simulink model "warplab_mimo_4x4"  (Simulink 6.5)
settings: Solver=ode45  StartTime=0.0  StopTime=20000  RelTol=1e-3
undefined symbols (not defined in the file): gcbh, xlBlockLoadCallback
libraries: xbsIndex_r4 x188
(part 4 of 17)

== system warplab_mimo_4x4/Radio_1 Tx_Buffer ==
  RdAddr : Inport
  Rst : Inport  Port=2
  En : Inport  Port=3
  Constant2_SMWOAddr_TxBuff_Radio1_SMWODataI_TxBuff_Radio1_SMWOWE_TxBuff_Radio1 : Constant  Value=0  OutDataType=sfix(16)  ConRadixGroup=Use specified scaling  OutScaling=2^0  SampleTime=inf  FramePeriod=inf
  Constant3 : S-Function  LoadFcn=xlBlockLoadCallback(gcbh);  FunctionName=sysgen  Parameters=ptable_  mask(Xilinx Constant Block Block){arith_type_sgadvanced=, arith_type=Unsigned, const=0, n_bits=32, bin_pt=0, explicit_period_sgadvanced=, explicit_period=off, period=1, dsp48_infoedit=The use of this block for DSP48 instructions is deprecated.  Please use the Opmode block., equ=P=C, opselect_sgadvanced=, opselect=C, inp2_sgadvanced=, inp2=PCIN>>17, opr_sgadvanced=, opr=+, inp1_sgadvanced=, inp1=P, carry_sgadvanced=, carry=CIN, dbl_ovrd_sgadvanced=, dbl_ovrd=off, has_advanced_control=0, sggui_pos=-1,-1,-1,-1, block_type=constant, block_version=VER_STRING_GOES_HERE, sg_icon_stat=25,18,0,1,white,blue,0,c7c04a0c, sg_mask_display=|, sg_list_contents=, sg_blockgui_xml=}
      mask sg_mask_display=|
      | fprintf('','COMMENT: begin icon graphics');
      | patch([0 55 55 0 ],[0 0 26 26 ],[0.77 0.82 0.91]);
      | patch([20 16 22 16 20 27 29 31 38 32 26 22 28 22 26 32 38 31 29 27 20 ],[3 7 13 19 23 23 21 23 23 17 23 19 13 7 3 9 3 3 5 3 3 ],[0.98 0.96 0.92]);
      | plot([0 0 55 55 0 ],[0 26 26 0 0 ]);
      | fprintf('','COMMENT: end icon graphics');
      | fprintf('','COMMENT: begin icon text');
      | color('black');port_label('output',1,'0');
      | fprintf('','COMMENT: end icon text');
      mask prompts: arith_type_sgadvanced ""; arith_type "Type"; const "Constant value"; n_bits "Number of bits"; bin_pt "Binary point"; explicit_period_sgadvanced ""; explicit_period "Sampled constant"; period "Sample period"; dsp48_infoedit ""; equ "DSP48 operation"; opselect_sgadvanced ""; opselect "Operation select"; inp2_sgadvanced ""; inp2 "Z mux"; opr_sgadvanced ""; opr "Operand"; inp1_sgadvanced ""; inp1 "YX muxes"; carry_sgadvanced ""; carry "Carry input"; dbl_ovrd_sgadvanced ""; dbl_ovrd "Override with doubles"; has_advanced_control ""; sggui_pos ""; block_type ""; block_version ""; sg_icon_stat ""; sg_mask_display ""; sg_list_contents ""; sg_blockgui_xml ""
      mask help: Xilinx Constant Block
      mask init: same as warplab_mimo_4x4/CaptureDone/zero3
      settings: CopyFcn=xlBlockMoveCallback(gcbh);  DeleteFcn=xlDestroyGui(gcbh);  ModelCloseFcn=xlDestroyGui(gcbh);  PreSaveFcn=xlBlockPreSaveCallback(gcbh);  PostSaveFcn=xlBlockPostSaveCallback(gcbh);  DestroyFcn=xlDestroyGui(gcbh);  OpenFcn=xlOpenGui(gcbh, 'constant_gui.xml', @constantenablement, @constantaction)  CloseFcn=xlDestroyGui(gcbh);  MoveFcn=xlBlockMoveCallback(gcbh);
      mask Help: eval('xlWeb(xlhtmldoclink(''Constant''))');
      mask StyleString: edit,popup(Boolean|Signed (2's comp)|Unsigned|DSP48 Instruction),edit,edit,edit,edit,checkbox,edit,edit,edit,edit,popup(C + A*B|PCIN + A*B|P + A*B|A * B|C + A:B|C - A:B|C|Custom),edit,popup(0|PCIN|P|C|PCIN>>17|P>>17),edit,popup(+|-),edit,popup(0|P|A:B|A*B|C|P+C|A:B+C),edit,popup(0|1|CIN|~SIGN(P or PCIN)|~SIGN(A*B or A:B)|~SIGND(A*B or A:B)),edit,checkbox,edit,edit,edit,edit,edit,edit,edit,edit
      mask Display:
      | fprintf('','COMMENT: begin icon graphics');
      | patch([0 55 55 0 ],[0 0 26 26 ],[0.77 0.82 0.91]);
      | patch([20 16 22 16 20 27 29 31 38 32 26 22 28 22 26 32 38 31 29 27 20 ],[3 7 13 19 23 23 21 23 23 17 23 19 13 7 3 9 3 3 5 3 3 ],[0.98 0.96 0.92]);
      | plot([0 0 55 55 0 ],[0 26 26 0 0 ]);
      | fprintf('','COMMENT: end icon graphics');
      | fprintf('','COMMENT: begin icon text');
      | color('black');port_label('output',1,'0');
      | fprintf('','COMMENT: end icon text');
  Constant4 : S-Function  LoadFcn=xlBlockLoadCallback(gcbh);  FunctionName=sysgen  Parameters=ptable_  mask(Xilinx Constant Block Block){arith_type_sgadvanced=, arith_type=Boolean, const=0, n_bits=1, bin_pt=0, explicit_period_sgadvanced=, explicit_period=off, period=1, dsp48_infoedit=The use of this block for DSP48 instructions is deprecated.  Please use the Opmode block., equ=P=C, opselect_sgadvanced=, opselect=C, inp2_sgadvanced=, inp2=PCIN>>17, opr_sgadvanced=, opr=+, inp1_sgadvanced=, inp1=P, carry_sgadvanced=, carry=CIN, dbl_ovrd_sgadvanced=, dbl_ovrd=off, has_advanced_control=0, sggui_pos=-1,-1,-1,-1, block_type=constant, block_version=VER_STRING_GOES_HERE, sg_icon_stat=25,18,0,1,white,blue,0,c7c04a0c, sg_mask_display=|, sg_list_contents=, sg_blockgui_xml=}
      mask sg_mask_display=|
      | fprintf('','COMMENT: begin icon graphics');
      | patch([0 55 55 0 ],[0 0 26 26 ],[0.77 0.82 0.91]);
      | patch([20 16 22 16 20 27 29 31 38 32 26 22 28 22 26 32 38 31 29 27 20 ],[3 7 13 19 23 23 21 23 23 17 23 19 13 7 3 9 3 3 5 3 3 ],[0.98 0.96 0.92]);
      | plot([0 0 55 55 0 ],[0 26 26 0 0 ]);
      | fprintf('','COMMENT: end icon graphics');
      | fprintf('','COMMENT: begin icon text');
      | color('black');port_label('output',1,'0');
      | fprintf('','COMMENT: end icon text');
      mask prompts: arith_type_sgadvanced ""; arith_type "Type"; const "Constant value"; n_bits "Number of bits"; bin_pt "Binary point"; explicit_period_sgadvanced ""; explicit_period "Sampled constant"; period "Sample period"; dsp48_infoedit ""; equ "DSP48 operation"; opselect_sgadvanced ""; opselect "Operation select"; inp2_sgadvanced ""; inp2 "Z mux"; opr_sgadvanced ""; opr "Operand"; inp1_sgadvanced ""; inp1 "YX muxes"; carry_sgadvanced ""; carry "Carry input"; dbl_ovrd_sgadvanced ""; dbl_ovrd "Override with doubles"; has_advanced_control ""; sggui_pos ""; block_type ""; block_version ""; sg_icon_stat ""; sg_mask_display ""; sg_list_contents ""; sg_blockgui_xml ""
      mask help: Xilinx Constant Block
      mask init: same as warplab_mimo_4x4/CaptureDone/zero3
      settings: CopyFcn=xlBlockMoveCallback(gcbh);  DeleteFcn=xlDestroyGui(gcbh);  ModelCloseFcn=xlDestroyGui(gcbh);  PreSaveFcn=xlBlockPreSaveCallback(gcbh);  PostSaveFcn=xlBlockPostSaveCallback(gcbh);  DestroyFcn=xlDestroyGui(gcbh);  OpenFcn=xlOpenGui(gcbh, 'constant_gui.xml', @constantenablement, @constantaction)  CloseFcn=xlDestroyGui(gcbh);  MoveFcn=xlBlockMoveCallback(gcbh);
      mask Help: eval('xlWeb(xlhtmldoclink(''Constant''))');
      mask StyleString: edit,popup(Boolean|Signed (2's comp)|Unsigned|DSP48 Instruction),edit,edit,edit,edit,checkbox,edit,edit,edit,edit,popup(C + A*B|PCIN + A*B|P + A*B|A * B|C + A:B|C - A:B|C|Custom),edit,popup(0|PCIN|P|C|PCIN>>17|P>>17),edit,popup(+|-),edit,popup(0|P|A:B|A*B|C|P+C|A:B+C),edit,popup(0|1|CIN|~SIGN(P or PCIN)|~SIGN(A*B or A:B)|~SIGND(A*B or A:B)),edit,checkbox,edit,edit,edit,edit,edit,edit,edit,edit
      mask Display:
      | fprintf('','COMMENT: begin icon graphics');
      | patch([0 55 55 0 ],[0 0 26 26 ],[0.77 0.82 0.91]);
      | patch([20 16 22 16 20 27 29 31 38 32 26 22 28 22 26 32 38 31 29 27 20 ],[3 7 13 19 23 23 21 23 23 17 23 19 13 7 3 9 3 3 5 3 3 ],[0.98 0.96 0.92]);
      | plot([0 0 55 55 0 ],[0 26 26 0 0 ]);
      | fprintf('','COMMENT: end icon graphics');
      | fprintf('','COMMENT: begin icon text');
      | color('black');port_label('output',1,'0');
      | fprintf('','COMMENT: end icon text');
  Convert : S-Function  LoadFcn=xlBlockLoadCallback(gcbh);  FunctionName=sysgen  Parameters=ptable_  mask(Xilinx Type Converter Block){infoedit=Hardware notes: rounding and saturating require hardware resources; truncating and wrapping do not., arith_type_sgadvanced=, arith_type=Boolean, n_bits=16, bin_pt=14, quantization_sgadvanced=, quantization=Truncate, overflow_sgadvanced=, overflow=Wrap, latency=0, dbl_ovrd_sgadvanced=, dbl_ovrd=off, pipeline_sgadvanced=, pipeline=off, xl_use_area_sgadvanced=, xl_use_area=off, xl_area=[0,0,0,0,0,0,0], has_advanced_control=0, sggui_pos=20,20,374,375, block_type=convert, block_version=8.2, sg_icon_stat=20,14,1,1,white,blue,0,0eb6e735, sg_mask_display=|, sg_list_contents=, sg_blockgui_xml=}
      mask sg_mask_display=|
      | fprintf('','COMMENT: begin icon graphics');
      | patch([0 20 20 0 ],[0 0 14 14 ],[0.77 0.82 0.91]);
      | patch([6 4 7 4 6 10 11 12 16 13 10 8 11 8 10 13 16 12 11 10 6 ],[2 4 7 10 12 12 11 12 12 9 12 10 7 4 2 5 2 2 3 2 2 ],[0.98 0.96 0.92]);
      | plot([0 0 20 20 0 ],[0 14 14 0 0 ]);
      | fprintf('','COMMENT: end icon graphics');
      | fprintf('','COMMENT: begin icon text');
      | color('black');port_label('output',1,'cast');
      | fprintf('','COMMENT: end icon text');
      mask prompts: infoedit ""; arith_type_sgadvanced ""; arith_type "Type"; n_bits "Number of bits"; bin_pt "Binary point"; quantization_sgadvanced ""; overflow_sgadvanced ""; dbl_ovrd_sgadvanced ""; dbl_ovrd "Override with doubles"; pipeline_sgadvanced ""; pipeline "Pipeline for maximum performance"; xl_use_area_sgadvanced ""; xl_use_area "Define FPGA area for resource estimation"; xl_area "FPGA area [slices, FFs, BRAMs, LUTs, IOBs, emb. mults, TBUFs]"; has_advanced_control ""; sggui_pos ""; block_type ""; block_version ""; sg_icon_stat ""; sg_mask_display ""; sg_list_contents ""; sg_blockgui_xml ""
      mask help: Hardware notes: rounding and saturating require hardware resources; truncating and wrapping do not.
      mask init: same as warplab_mimo_4x4/Mem_Control/Convert1
      settings: CopyFcn=xlBlockMoveCallback(gcbh);  DeleteFcn=xlDestroyGui(gcbh);  ModelCloseFcn=xlDestroyGui(gcbh);  PreSaveFcn=xlBlockPreSaveCallback(gcbh);  PostSaveFcn=xlBlockPostSaveCallback(gcbh);  DestroyFcn=xlDestroyGui(gcbh);  OpenFcn=xlOpenGui(gcbh, 'convert_gui.xml', @convertenablement, -1)  CloseFcn=xlDestroyGui(gcbh);  MoveFcn=xlBlockMoveCallback(gcbh);
      mask Help: eval('xlWeb(xlhtmldoclink(''Convert''))');
      mask StyleString: edit,edit,popup(Boolean|Signed  (2's comp)|Unsigned),edit,edit,edit,popup(Truncate|Round  (unbiased: +/- Inf)|Round  (unbiased: Even Values)),edit,popup(Wrap|Saturate|Flag as error),edit,edit,checkbox,edit,checkbox,edit,checkbox,edit,edit,edit,edit,edit,edit,edit,edit,edit
      mask Display:
      | fprintf('','COMMENT: begin icon graphics');
      | patch([0 20 20 0 ],[0 0 14 14 ],[0.77 0.82 0.91]);
      | patch([6 4 7 4 6 10 11 12 16 13 10 8 11 8 10 13 16 12 11 10 6 ],[2 4 7 10 12 12 11 12 12 9 12 10 7 4 2 5 2 2 3 2 2 ],[0.98 0.96 0.92]);
      | plot([0 0 20 20 0 ],[0 14 14 0 0 ]);
      | fprintf('','COMMENT: end icon graphics');
      | fprintf('','COMMENT: begin icon text');
      | color('black');port_label('output',1,'cast');
      | fprintf('','COMMENT: end icon text');
  Inverter : S-Function  LoadFcn=xlBlockLoadCallback(gcbh);  FunctionName=sysgen  Parameters=ptable_  mask(Xilinx Inverter Block){infoedit=Bitwise logical negation (one's complement) operator., en_sgadvanced=, en=off, latency=0, dbl_ovrd_sgadvanced=, dbl_ovrd=off, xl_use_area_sgadvanced=, xl_use_area=off, xl_area=[0,0,0,0,0,0,0], has_advanced_control=0, sggui_pos=-1,-1,-1,-1, block_type=inv, block_version=9.1.01, sg_icon_stat=30,18,1,1,white,blue,0,1ab4a85f, sg_mask_display=|, sg_list_contents=, sg_blockgui_xml=}
      mask sg_mask_display=|
      | fprintf('','COMMENT: begin icon graphics');
      | patch([0 30 30 0 ],[0 0 18 18 ],[0.77 0.82 0.91]);
      | patch([10 7 11 7 10 15 16 17 22 18 14 11 15 11 14 18 22 17 16 15 10 ],[2 5 9 13 16 16 15 16 16 12 16 13 9 5 2 6 2 2 3 2 2 ],[0.98 0.96 0.92]);
      | plot([0 0 30 30 0 ],[0 18 18 0 0 ]);
      | fprintf('','COMMENT: end icon graphics');
      | fprintf('','COMMENT: begin icon text');
      | color('black');disp('not');
      | fprintf('','COMMENT: end icon text');
      mask prompts: infoedit ""; en_sgadvanced ""; en "Provide enable port"; dbl_ovrd_sgadvanced ""; dbl_ovrd "Override with doubles"; xl_use_area_sgadvanced ""; xl_use_area "Define FPGA area for resource estimation"; xl_area "FPGA area [slices, FFs, BRAMs, LUTs, IOBs, emb. mults, TBUFs]"; has_advanced_control ""; sggui_pos ""; block_type ""; block_version ""; sg_icon_stat ""; sg_mask_display ""; sg_list_contents ""; sg_blockgui_xml ""
      mask help: Bitwise logical negation (one's complement) operator.
      mask init: same as warplab_mimo_4x4/Inverter
      settings: CopyFcn=xlBlockMoveCallback(gcbh);  DeleteFcn=xlDestroyGui(gcbh);  ModelCloseFcn=xlDestroyGui(gcbh);  PreSaveFcn=xlBlockPreSaveCallback(gcbh);  PostSaveFcn=xlBlockPostSaveCallback(gcbh);  DestroyFcn=xlDestroyGui(gcbh);  OpenFcn=xlOpenGui(gcbh, 'inv_gui.xml', @xlmagicenablement, -1)  CloseFcn=xlDestroyGui(gcbh);  MoveFcn=xlBlockMoveCallback(gcbh);
      mask Help: eval('xlWeb(xlhtmldoclink(''Inverter''))');
      mask Display:
      | fprintf('','COMMENT: begin icon graphics');
      | patch([0 30 30 0 ],[0 0 18 18 ],[0.77 0.82 0.91]);
      | patch([10 7 11 7 10 15 16 17 22 18 14 11 15 11 14 18 22 17 16 15 10 ],[2 5 9 13 16 16 15 16 16 12 16 13 9 5 2 6 2 2 3 2 2 ],[0.98 0.96 0.92]);
      | plot([0 0 30 30 0 ],[0 18 18 0 0 ]);
      | fprintf('','COMMENT: end icon graphics');
      | fprintf('','COMMENT: begin icon text');
      | color('black');disp('not');
      | fprintf('','COMMENT: end icon text');
  Logical : S-Function  LoadFcn=xlBlockLoadCallback(gcbh);  FunctionName=sysgen  Parameters=ptable_  mask(Xilinx Logical Block Block){logical_function_sgadvanced=, logical_function=OR, inputs=2, en_sgadvanced=, en=off, latency=0, precision_sgadvanced=, precision=Full, arith_type_sgadvanced=, arith_type=Unsigned, n_bits=16, bin_pt=0, align_bp_sgadvanced=, align_bp=on, dbl_ovrd_sgadvanced=, dbl_ovrd=off, xl_use_area_sgadvanced=, xl_use_area=off, xl_area=[0,0,0,0,0,0,0], overflow=, quantization=, has_advanced_control=0, sggui_pos=-1,-1,-1,-1, block_type=logical, block_version=9.1.01, sg_icon_stat=55,60,2,1,white,blue,0,f4a65842, sg_mask_display=|, sg_list_contents=, sg_blockgui_xml=}
      mask sg_mask_display=|
      | fprintf('','COMMENT: begin icon graphics');
      | patch([0 55 55 0 ],[0 0 60 60 ],[0.77 0.82 0.91]);
      | patch([13 4 17 4 13 28 32 36 52 40 28 19 32 19 28 40 52 36 32 28 13 ],[8 17 30 43 52 52 48 52 52 40 52 43 30 17 8 20 8 8 12 8 8 ],[0.98 0.96 0.92]);
      | plot([0 0 55 55 0 ],[0 60 60 0 0 ]);
      | fprintf('','COMMENT: end icon graphics');
      | fprintf('','COMMENT: begin icon text');
      | color('black');disp('\newlineor\newlinez^{-0}','texmode','on');
      | fprintf('','COMMENT: end icon text');
      mask prompts: logical_function_sgadvanced ""; logical_function "Logical function"; inputs "Number of inputs"; en_sgadvanced ""; en "Provide enable port"; precision_sgadvanced ""; arith_type_sgadvanced ""; arith_type "Output Type"; n_bits "Number of bits"; bin_pt "Binary point"; align_bp_sgadvanced ""; align_bp "Align binary point"; dbl_ovrd_sgadvanced ""; dbl_ovrd "Override with doubles"; xl_use_area_sgadvanced ""; xl_use_area "Define FPGA area for resource estimation"; xl_area "FPGA area [slices, FFs, BRAMs, LUTs, IOBs, emb. mults, TBUFs]"; overflow ""; quantization ""; has_advanced_control ""; sggui_pos ""; block_type ""; block_version ""; sg_icon_stat ""; sg_mask_display ""; sg_list_contents ""; sg_blockgui_xml ""
      mask help: Xilinx Logical Block
      mask init: same as warplab_mimo_4x4/Logical
      settings: CopyFcn=xlBlockMoveCallback(gcbh);  DeleteFcn=xlDestroyGui(gcbh);  ModelCloseFcn=xlDestroyGui(gcbh);  PreSaveFcn=xlBlockPreSaveCallback(gcbh);  PostSaveFcn=xlBlockPostSaveCallback(gcbh);  DestroyFcn=xlDestroyGui(gcbh);  OpenFcn=xlOpenGui(gcbh, 'logical_gui.xml', @logicalenablement, -1)  CloseFcn=xlDestroyGui(gcbh);  MoveFcn=xlBlockMoveCallback(gcbh);
      mask Help: eval('xlWeb(xlhtmldoclink(''Logical''))');
      mask StyleString: edit,popup(AND|NAND|OR|NOR|XOR|XNOR),edit,edit,checkbox,edit,edit,popup(Full|User Defined),edit,popup(Signed  (2's comp)|Unsigned),edit,edit,edit,checkbox,edit,checkbox,edit,checkbox,edit,edit,edit,edit,edit,edit,edit,edit,edit,edit,edit
      mask Display:
      | fprintf('','COMMENT: begin icon graphics');
      | patch([0 55 55 0 ],[0 0 60 60 ],[0.77 0.82 0.91]);
      | patch([13 4 17 4 13 28 32 36 52 40 28 19 32 19 28 40 52 36 32 28 13 ],[8 17 30 43 52 52 48 52 52 40 52 43 30 17 8 20 8 8 12 8 8 ],[0.98 0.96 0.92]);
      | plot([0 0 55 55 0 ],[0 60 60 0 0 ]);
      | fprintf('','COMMENT: end icon graphics');
      | fprintf('','COMMENT: begin icon text');
      | color('black');disp('\newlineor\newlinez^{-0}','texmode','on');
      | fprintf('','COMMENT: end icon text');
  SMWOAddr_TxBuff_Radio1_slice_sm2 : xbsIndex_r4/Slice  nbits=14  boolean_output=off  mode=Lower Bit Location + Width  bit1=0  base1=MSB of Input  bit0=0  base0=LSB of Input  dbl_ovrd=off  block_type=slice
      settings: infoedit="Extracts a given range of bits from each input sample and presents it at the output.  The output type is ordinarily unsigned with binary point at zero, but can be Boolean when the slice is one bit wide.<P><P>Hardware notes: In hardware this block costs nothing."  block_version=VER_STRING_GOES_HERE
  SMWODataI_TxBuff_Radio1_force_sm2 : xbsIndex_r4/Reinterpret  force_arith_type=on  arith_type=Unsigned  force_bin_pt=off  bin_pt=0  block_type=cast
      settings: infoedit="Changes type of samples without altering their binary representation.<P><P>Hardware notes: In hardware this block costs nothing.<P><P>Example:  Suppose the input is 6 bits wide, signed, with 2 fractional bits, and the output is forced to unsigned with 0 fractional bits.  Then an input of -2.0 (1110.00 in binary 2's complement) becomes an output of 56 (111000 in binary)."  block_version=VER_STRING_GOES_HERE
  SMWO_TxBuff_Radio1 : S-Function  LoadFcn=xlBlockLoadCallback(gcbh);  FunctionName=sysgen  Parameters=ptable_  mask(Xilinx Dual Port Random Access Memory Block){depth=2^14, initVector=1:2^14, distributed_mem_sgadvanced=, distributed_mem=Block RAM, init_a=0, init_b=0, rst_a_sgadvanced=, rst_a=on, rst_b_sgadvanced=, rst_b=off, en_a_sgadvanced=, en_a=off, en_b_sgadvanced=, en_b=off, latency=1, write_mode_A_sgadvanced=, write_mode_A=Read After Write, write_mode_B_sgadvanced=, write_mode_B=Read After Write, dbl_ovrd_sgadvanced=, dbl_ovrd=off, optimize_sgadvanced=, optimize=Area, use_rpm_sgadvanced=, use_rpm=on, xl_use_area_sgadvanced=, xl_use_area=off, xl_area=[0,0,0,0,0,0,0], explicit_period=, period=, infoedit=, has_advanced_control=0, sggui_pos=-1,-1,-1,-1, block_type=dpram, block_version=VER_STRING_GOES_HERE, sg_icon_stat=90,288,7,2,white,blue,0,9e97e038, sg_mask_display=|, sg_list_contents=, sg_blockgui_xml=}
      mask sg_mask_display=|
      | fprintf('','COMMENT: begin icon graphics ');
      | patch([0 90 90 0 ],[0 0 288 288 ],[0.77 0.82 0.91]);
      | patch([21 6 27 6 21 45 51 57 82 62 43 29 50 29 43 62 82 57 51 45 21 ],[109 124 145 166 181 181 175 181 181 161 180 166 145 124 110 129 109 109 115 109 109 ],[0.98 0.96 0.92]);
      | plot([0 0 90 90 0 ],[0 288 288 0 0 ]);
      | fprintf('','COMMENT: end icon graphics');
      | fprintf('','COMMENT: begin icon text ');
      | color('black');port_label('input',1,'addra');
      | color('black');port_label('input',2,'dina');
      | color('black');port_label('input',3,'wea');
      | color('black');port_label('input',4,'addrb');
      | color('black');port_label('input',5,'dinb');
      | color('black');port_label('input',6,'web');
      | color('black');port_label('input',7,'rsta');
      | color('black');port_label('output',1,'A');
      | color('black');port_label('output',2,'B');
      | fprintf('','COMMENT: end icon text');
      mask prompts: initVector "Initial value vector"; distributed_mem_sgadvanced ""; distributed_mem "Memory Type"; init_a "Initial value for port <tt>A</tt> output register"; init_b "Initial value for port <tt>B</tt> output register"; rst_a_sgadvanced ""; rst_a "Provide synchronous reset port for port <tt>A</tt> output register"; rst_b_sgadvanced ""; rst_b "Provide synchronous reset port for port <tt>B</tt> output register"; en_a_sgadvanced ""; en_a "Provide enable port for port <tt>A</tt>"; en_b_sgadvanced ""; en_b "Provide enable port for port <tt>B</tt>"; write_mode_A_sgadvanced ""; write_mode_A "Port <tt>A</tt>"; write_mode_B_sgadvanced ""; write_mode_B "Port <tt>B</tt>"; dbl_ovrd_sgadvanced ""; dbl_ovrd "Override with doubles"; optimize_sgadvanced ""; optimize "Optimize for"; use_rpm_sgadvanced ""; use_rpm "Use core placement information"; xl_use_area_sgadvanced ""; xl_use_area "Define FPGA area for resource estimation"; xl_area "FPGA area [slices, FFs, BRAMs, LUTs, IOBs, emb. mults, TBUFs]"; explicit_period ""; period ""; infoedit ""; has_advanced_control ""; sggui_pos ""; block_type ""; block_version ""; sg_icon_stat ""; sg_mask_display ""; sg_list_contents ""; sg_blockgui_xml ""
      mask help: Xilinx Dual Port Random Access Memory
      mask init: same as warplab_mimo_4x4/Radio_1 Rx_Buffers/SMRO_RxBuff_Radio1
      settings: CopyFcn=xlBlockMoveCallback(gcbh);  DeleteFcn=xlDestroyGui(gcbh);  ModelCloseFcn=xlDestroyGui(gcbh);  PreSaveFcn=xlBlockPreSaveCallback(gcbh);  PostSaveFcn=xlBlockPostSaveCallback(gcbh);  DestroyFcn=xlDestroyGui(gcbh);  OpenFcn=xlOpenGui(gcbh, 'dpram_gui.xml', @dpramenablement, -1)  CloseFcn=xlDestroyGui(gcbh);  MoveFcn=xlBlockMoveCallback(gcbh);
      mask Help: eval('xlWeb(xlhtmldoclink(''Dual Port RAM''))');
      mask StyleString: edit,edit,edit,popup(Distributed memory|Block RAM),edit,edit,edit,checkbox,edit,checkbox,edit,checkbox,edit,checkbox,edit,edit,popup(Read After Write|Read Before Write|No Read On Write),edit,popup(Read After Write|Read Before Write|No Read On Write),edit,checkbox,edit,popup(Area|Speed),edit,checkbox,edit,checkbox,edit,edit,edit,edit,edit,edit,edit,edit,edit,edit,edit,edit
      mask Display:
      | fprintf('','COMMENT: begin icon graphics ');
      | patch([0 90 90 0 ],[0 0 288 288 ],[0.77 0.82 0.91]);
      | patch([21 6 27 6 21 45 51 57 82 62 43 29 50 29 43 62 82 57 51 45 21 ],[109 124 145 166 181 181 175 181 181 161 180 166 145 124 110 129 109 109 115 109 109 ],[0.98 0.96 0.92]);
      | plot([0 0 90 90 0 ],[0 288 288 0 0 ]);
      | fprintf('','COMMENT: end icon graphics');
      | fprintf('','COMMENT: begin icon text ');
      | color('black');port_label('input',1,'addra');
      | color('black');port_label('input',2,'dina');
      | color('black');port_label('input',3,'wea');
      | color('black');port_label('input',4,'addrb');
      | color('black');port_label('input',5,'dinb');
      | color('black');port_label('input',6,'web');
      | color('black');port_label('input',7,'rsta');
      | color('black');port_label('output',1,'A');
      | color('black');port_label('output',2,'B');
      | fprintf('','COMMENT: end icon text');
  Terminator1 : Terminator
  Data : Outport
  wires:
  SMWO_TxBuff_Radio1/2 -> Terminator1/1
  Constant3/1 -> SMWO_TxBuff_Radio1/2
  Constant4/1 -> SMWO_TxBuff_Radio1/3
  RdAddr/1 -> SMWO_TxBuff_Radio1/1
  SMWO_TxBuff_Radio1/1 -> Data/1
  Logical/1 -> SMWO_TxBuff_Radio1/7
  Rst/1 -> Logical/1
  Inverter/1 -> Logical/2
  En/1 -> Convert/1
  Convert/1 -> Inverter/1
  [SMWOAddr_0] -> SMWOAddr_TxBuff_Radio1_slice_sm2/1
  SMWOAddr_TxBuff_Radio1_slice_sm2/1 -> SMWO_TxBuff_Radio1/4
  [SMWODataI_0] -> SMWODataI_TxBuff_Radio1_force_sm2/1
  SMWODataI_TxBuff_Radio1_force_sm2/1 -> SMWO_TxBuff_Radio1/5
  [SMWOWE_0] -> SMWO_TxBuff_Radio1/6

== system warplab_mimo_4x4/Radio_1_Inputs ==
  ADC_I : Subsystem
  ADC_Q : Subsystem
  Concatenates_1 : Subsystem
  Scope : Scope  NumInputPorts=3
      settings: YMin=-5~-5~-5  YMax=5~5~5
  Radio 1 I/Q : Outport
  wires:
  ADC_Q/2(ADC Q) -> Concatenates_1/4(ADC_Q), Scope/2
  ADC_Q/1(OTR Q) -> Concatenates_1/3(OTR_Q)
  ADC_I/2(ADC I) -> Concatenates_1/2(ADC_I), Scope/1
  ADC_I/1(OTR I) -> Concatenates_1/1(OTR_I)
  Concatenates_1/1(32b) -> Radio 1 I/Q/1

== system warplab_mimo_4x4/Radio_1_Outputs ==
  32b : Inport
  16LSB : S-Function  LoadFcn=xlBlockLoadCallback(gcbh);  FunctionName=sysgen  Parameters=ptable_  mask(Xilinx Bit Slice Extractor Block){infoedit=Extracts a given range of bits from each input sample and presents it at the output.  The output type is ordinarily unsigned with binary point at zero, but can be Boolean when the slice is one bit wide.<P><P>Hardware notes: In hardware this block costs nothing., nbits=16, boolean_output_sgadvanced=, boolean_output=off, mode_sgadvanced=, mode=Lower Bit Location + Width, bit1=0, base1_sgadvanced=, base1=MSB of Input, bit0=0, base0_sgadvanced=, base0=LSB of Input, dbl_ovrd_sgadvanced=, dbl_ovrd=off, has_advanced_control=0, sggui_pos=20,20,442,407, block_type=slice, block_version=8.2, sg_icon_stat=40,16,1,1,white,blue,0,fe24a11e, sg_mask_display=|, sg_list_contents=, sg_blockgui_xml=}
      mask sg_mask_display=|
      | fprintf('','COMMENT: begin icon graphics');
      | patch([0 40 40 0 ],[0 0 16 16 ],[0.77 0.82 0.91]);
      | patch([16 13 17 13 16 20 21 22 27 23 20 18 22 18 20 23 27 22 21 20 16 ],[2 5 9 13 16 16 15 16 16 12 15 13 9 5 3 6 2 2 3 2 2 ],[0.98 0.96 0.92]);
      | plot([0 0 40 40 0 ],[0 16 16 0 0 ]);
      | fprintf('','COMMENT: end icon graphics');
      | fprintf('','COMMENT: begin icon text');
      | color('black');port_label('output',1,'[a:b]');
      | fprintf('','COMMENT: end icon text');
      mask prompts: infoedit ""; nbits "Width of slice (number of bits)"; boolean_output_sgadvanced ""; boolean_output "Boolean output"; mode_sgadvanced ""; mode "Specify range as"; bit1 "Offset of top bit"; base1_sgadvanced ""; base1 "Relative to"; bit0 "Offset of bottom bit"; base0_sgadvanced ""; base0 "Relative to"; dbl_ovrd_sgadvanced ""; dbl_ovrd "Override with doubles"; has_advanced_control ""; sggui_pos ""; block_type ""; block_version ""; sg_icon_stat ""; sg_mask_display ""; sg_list_contents ""; sg_blockgui_xml ""
      mask help:
      | Extracts a given range of bits from each input sample and presents it at the output.  The output type is ordinarily unsigned with binary point at zero, but can be Boolean when the slice is one bit wide.
      |
      | Hardware notes: In hardware this block costs nothing.
      mask init:
      | try
      |   tmp_gcb = gcb;
      |   tmp_gcbh = gcbh;
      |   xlMungeMaskParams;
      |   block_config = 'sysgen_blockset:Slice_config';
      |   serialized_declarations = '{''base0''=>''Int'',''base1''=>''Int'',''bit0''=>''Int'',''bit1''=>''Int'',''boolean_output''=>''Int'',''mode''=>''Int'',''nbits''=>''Int'',''sim_engine''=>''Int'',''sysgen_root''=>''String''}';
      |   xlslice_init();
      |   ptable_ = xlblockprep(get_param(tmp_gcb, 'MaskWSVariables'));
      | catch
      |   global dbgsysgen;
      |   if(~isempty(dbgsysgen) && dbgsysgen)
      |     e = regexprep(lasterr, '\n', '\nError: ');
      |     disp(['Error: While running MaskInit code on block ' tmp_gcb ': ' e]);
      |     error(e);
      |   end
      | end
      settings: CopyFcn=xlBlockMoveCallback(gcbh);  DeleteFcn=xlDestroyGui(gcbh);  ModelCloseFcn=xlDestroyGui(gcbh);  PreSaveFcn=xlBlockPreSaveCallback(gcbh);  PostSaveFcn=xlBlockPostSaveCallback(gcbh);  DestroyFcn=xlDestroyGui(gcbh);  OpenFcn=xlOpenGui(gcbh, 'slice_gui.xml', @sliceenablement, -1)  CloseFcn=xlDestroyGui(gcbh);  MoveFcn=xlBlockMoveCallback(gcbh);
      mask Help: eval('xlWeb(xlhtmldoclink(''Slice''))');
      mask StyleString: edit,edit,edit,checkbox,edit,popup(Two Bit Locations|Upper Bit Location + Width|Lower Bit Location + Width),edit,edit,popup(LSB of Input|Binary Point of Input|MSB of Input),edit,edit,popup(LSB of Input|Binary Point of Input|MSB of Input),edit,checkbox,edit,edit,edit,edit,edit,edit,edit,edit
      mask Display:
      | fprintf('','COMMENT: begin icon graphics');
      | patch([0 40 40 0 ],[0 0 16 16 ],[0.77 0.82 0.91]);
      | patch([16 13 17 13 16 20 21 22 27 23 20 18 22 18 20 23 27 22 21 20 16 ],[2 5 9 13 16 16 15 16 16 12 15 13 9 5 3 6 2 2 3 2 2 ],[0.98 0.96 0.92]);
      | plot([0 0 40 40 0 ],[0 16 16 0 0 ]);
      | fprintf('','COMMENT: end icon graphics');
      | fprintf('','COMMENT: begin icon text');
      | color('black');port_label('output',1,'[a:b]');
      | fprintf('','COMMENT: end icon text');
  16MSB : S-Function  LoadFcn=xlBlockLoadCallback(gcbh);  FunctionName=sysgen  Parameters=ptable_  mask(Xilinx Bit Slice Extractor Block){infoedit=Extracts a given range of bits from each input sample and presents it at the output.  The output type is ordinarily unsigned with binary point at zero, but can be Boolean when the slice is one bit wide.<P><P>Hardware notes: In hardware this block costs nothing., nbits=16, boolean_output_sgadvanced=, boolean_output=off, mode_sgadvanced=, mode=Upper Bit Location + Width, bit1=0, base1_sgadvanced=, base1=MSB of Input, bit0=0, base0_sgadvanced=, base0=LSB of Input, dbl_ovrd_sgadvanced=, dbl_ovrd=off, has_advanced_control=0, sggui_pos=20,20,442,407, block_type=slice, block_version=8.2, sg_icon_stat=40,18,1,1,white,blue,0,fe24a11e, sg_mask_display=|, sg_list_contents=, sg_blockgui_xml=}
      mask sg_mask_display=|
      | fprintf('','COMMENT: begin icon graphics');
      | patch([0 40 40 0 ],[0 0 18 18 ],[0.77 0.82 0.91]);
      | patch([15 12 16 12 15 20 21 22 27 23 19 16 20 16 19 23 27 22 21 20 15 ],[2 5 9 13 16 16 15 16 16 12 16 13 9 5 2 6 2 2 3 2 2 ],[0.98 0.96 0.92]);
      | plot([0 0 40 40 0 ],[0 18 18 0 0 ]);
      | fprintf('','COMMENT: end icon graphics');
      | fprintf('','COMMENT: begin icon text');
      | color('black');port_label('output',1,'[a:b]');
      | fprintf('','COMMENT: end icon text');
      mask prompts: infoedit ""; nbits "Width of slice (number of bits)"; boolean_output_sgadvanced ""; boolean_output "Boolean output"; mode_sgadvanced ""; mode "Specify range as"; bit1 "Offset of top bit"; base1_sgadvanced ""; base1 "Relative to"; bit0 "Offset of bottom bit"; base0_sgadvanced ""; base0 "Relative to"; dbl_ovrd_sgadvanced ""; dbl_ovrd "Override with doubles"; has_advanced_control ""; sggui_pos ""; block_type ""; block_version ""; sg_icon_stat ""; sg_mask_display ""; sg_list_contents ""; sg_blockgui_xml ""
      mask help:
      | Extracts a given range of bits from each input sample and presents it at the output.  The output type is ordinarily unsigned with binary point at zero, but can be Boolean when the slice is one bit wide.
      |
      | Hardware notes: In hardware this block costs nothing.
      mask init: same as warplab_mimo_4x4/Radio_1_Outputs/16LSB
      settings: CopyFcn=xlBlockMoveCallback(gcbh);  DeleteFcn=xlDestroyGui(gcbh);  ModelCloseFcn=xlDestroyGui(gcbh);  PreSaveFcn=xlBlockPreSaveCallback(gcbh);  PostSaveFcn=xlBlockPostSaveCallback(gcbh);  DestroyFcn=xlDestroyGui(gcbh);  OpenFcn=xlOpenGui(gcbh, 'slice_gui.xml', @sliceenablement, -1)  CloseFcn=xlDestroyGui(gcbh);  MoveFcn=xlBlockMoveCallback(gcbh);
      mask Help: eval('xlWeb(xlhtmldoclink(''Slice''))');
      mask StyleString: edit,edit,edit,checkbox,edit,popup(Two Bit Locations|Upper Bit Location + Width|Lower Bit Location + Width),edit,edit,popup(LSB of Input|Binary Point of Input|MSB of Input),edit,edit,popup(LSB of Input|Binary Point of Input|MSB of Input),edit,checkbox,edit,edit,edit,edit,edit,edit,edit,edit
      mask Display:
      | fprintf('','COMMENT: begin icon graphics');
      | patch([0 40 40 0 ],[0 0 18 18 ],[0.77 0.82 0.91]);
      | patch([15 12 16 12 15 20 21 22 27 23 19 16 20 16 19 23 27 22 21 20 15 ],[2 5 9 13 16 16 15 16 16 12 16 13 9 5 2 6 2 2 3 2 2 ],[0.98 0.96 0.92]);
      | plot([0 0 40 40 0 ],[0 18 18 0 0 ]);
      | fprintf('','COMMENT: end icon graphics');
      | fprintf('','COMMENT: begin icon text');
      | color('black');port_label('output',1,'[a:b]');
      | fprintf('','COMMENT: end icon text');
  Radio_1_DAC_I : Subsystem
      mask Description: WARP Radio Board #1 I-channel DAC
      mask Display: image(imread('WARP_Logo.jpg'))
  Radio_1_DAC_Q : Subsystem
      mask Description: WARP Radio Board #1Q-channel DAC
      mask Display: image(imread('WARP_Logo.jpg'))
  Register : S-Function  LoadFcn=xlBlockLoadCallback(gcbh);  FunctionName=sysgen  Parameters=ptable_  mask(Xilinx Register Block){init=0, rst_sgadvanced=, rst=off, en_sgadvanced=, en=off, dbl_ovrd_sgadvanced=, dbl_ovrd=off, xl_use_area_sgadvanced=, xl_use_area=off, xl_area=[0,0,0,0,0,0,0], has_advanced_control=0, sggui_pos=-1,-1,-1,-1, block_type=register, block_version=8.2, sg_icon_stat=35,28,1,1,white,blue,0,ac6b57db, sg_mask_display=|, sg_list_contents=, sg_blockgui_xml=}
      mask sg_mask_display=|
      | fprintf('','COMMENT: begin icon graphics');
      | patch([0 35 35 0 ],[0 0 28 28 ],[0.77 0.82 0.91]);
      | patch([10 5 12 5 10 17 19 21 29 23 17 13 21 13 17 23 29 21 19 17 10 ],[3 8 15 22 27 27 25 27 27 21 27 23 15 7 3 9 3 3 5 3 3 ],[0.98 0.96 0.92]);
      | plot([0 0 35 35 0 ],[0 28 28 0 0 ]);
      | fprintf('','COMMENT: end icon graphics');
      | fprintf('','COMMENT: begin icon text');
      | color('black');port_label('input',1,'d');
      | color('black');port_label('output',1,'q');
      | color('black');disp('\bf{z^{-1}}','texmode','on');
      | fprintf('','COMMENT: end icon text');
      mask prompts: init "Initial value"; rst_sgadvanced ""; rst "Provide synchronous reset port"; en_sgadvanced ""; en "Provide enable port"; dbl_ovrd_sgadvanced ""; dbl_ovrd "Override with doubles"; xl_use_area_sgadvanced ""; xl_use_area "Define FPGA area for resource estimation"; xl_area "FPGA area [slices, FFs, BRAMs, LUTs, IOBs, emb. mults, TBUFs]"; has_advanced_control ""; sggui_pos ""; block_type ""; block_version ""; sg_icon_stat ""; sg_mask_display ""; sg_list_contents ""; sg_blockgui_xml ""
      mask help: Xilinx Register
      mask init: same as warplab_mimo_4x4/Mem_Control/Register
      settings: CopyFcn=xlBlockMoveCallback(gcbh);  DeleteFcn=xlDestroyGui(gcbh);  ModelCloseFcn=xlDestroyGui(gcbh);  PreSaveFcn=xlBlockPreSaveCallback(gcbh);  PostSaveFcn=xlBlockPostSaveCallback(gcbh);  DestroyFcn=xlDestroyGui(gcbh);  OpenFcn=xlOpenGui(gcbh, 'register_gui.xml', @xlmagicenablement, -1)  CloseFcn=xlDestroyGui(gcbh);  MoveFcn=xlBlockMoveCallback(gcbh);
      mask Help: eval('xlWeb(xlhtmldoclink(''Register''))');
      mask Display:
      | fprintf('','COMMENT: begin icon graphics');
      | patch([0 35 35 0 ],[0 0 28 28 ],[0.77 0.82 0.91]);
      | patch([10 5 12 5 10 17 19 21 29 23 17 13 21 13 17 23 29 21 19 17 10 ],[3 8 15 22 27 27 25 27 27 21 27 23 15 7 3 9 3 3 5 3 3 ],[0.98 0.96 0.92]);
      | plot([0 0 35 35 0 ],[0 28 28 0 0 ]);
      | fprintf('','COMMENT: end icon graphics');
      | fprintf('','COMMENT: begin icon text');
      | color('black');port_label('input',1,'d');
      | color('black');port_label('output',1,'q');
      | color('black');disp('\bf{z^{-1}}','texmode','on');
      | fprintf('','COMMENT: end icon text');
  Register1 : S-Function  LoadFcn=xlBlockLoadCallback(gcbh);  FunctionName=sysgen  Parameters=ptable_  mask(Xilinx Register Block){init=0, rst_sgadvanced=, rst=off, en_sgadvanced=, en=off, dbl_ovrd_sgadvanced=, dbl_ovrd=off, xl_use_area_sgadvanced=, xl_use_area=off, xl_area=[0,0,0,0,0,0,0], has_advanced_control=0, sggui_pos=-1,-1,-1,-1, block_type=register, block_version=8.2, sg_icon_stat=35,28,1,1,white,blue,0,ac6b57db, sg_mask_display=|, sg_list_contents=, sg_blockgui_xml=}
      mask sg_mask_display=|
      | fprintf('','COMMENT: begin icon graphics');
      | patch([0 35 35 0 ],[0 0 28 28 ],[0.77 0.82 0.91]);
      | patch([10 5 12 5 10 17 19 21 29 23 17 13 21 13 17 23 29 21 19 17 10 ],[3 8 15 22 27 27 25 27 27 21 27 23 15 7 3 9 3 3 5 3 3 ],[0.98 0.96 0.92]);
      | plot([0 0 35 35 0 ],[0 28 28 0 0 ]);
      | fprintf('','COMMENT: end icon graphics');
      | fprintf('','COMMENT: begin icon text');
      | color('black');port_label('input',1,'d');
      | color('black');port_label('output',1,'q');
      | color('black');disp('\bf{z^{-1}}','texmode','on');
      | fprintf('','COMMENT: end icon text');
      mask prompts: init "Initial value"; rst_sgadvanced ""; rst "Provide synchronous reset port"; en_sgadvanced ""; en "Provide enable port"; dbl_ovrd_sgadvanced ""; dbl_ovrd "Override with doubles"; xl_use_area_sgadvanced ""; xl_use_area "Define FPGA area for resource estimation"; xl_area "FPGA area [slices, FFs, BRAMs, LUTs, IOBs, emb. mults, TBUFs]"; has_advanced_control ""; sggui_pos ""; block_type ""; block_version ""; sg_icon_stat ""; sg_mask_display ""; sg_list_contents ""; sg_blockgui_xml ""
      mask help: Xilinx Register
      mask init: same as warplab_mimo_4x4/Mem_Control/Register
      settings: CopyFcn=xlBlockMoveCallback(gcbh);  DeleteFcn=xlDestroyGui(gcbh);  ModelCloseFcn=xlDestroyGui(gcbh);  PreSaveFcn=xlBlockPreSaveCallback(gcbh);  PostSaveFcn=xlBlockPostSaveCallback(gcbh);  DestroyFcn=xlDestroyGui(gcbh);  OpenFcn=xlOpenGui(gcbh, 'register_gui.xml', @xlmagicenablement, -1)  CloseFcn=xlDestroyGui(gcbh);  MoveFcn=xlBlockMoveCallback(gcbh);
      mask Help: eval('xlWeb(xlhtmldoclink(''Register''))');
      mask Display:
      | fprintf('','COMMENT: begin icon graphics');
      | patch([0 35 35 0 ],[0 0 28 28 ],[0.77 0.82 0.91]);
      | patch([10 5 12 5 10 17 19 21 29 23 17 13 21 13 17 23 29 21 19 17 10 ],[3 8 15 22 27 27 25 27 27 21 27 23 15 7 3 9 3 3 5 3 3 ],[0.98 0.96 0.92]);
      | plot([0 0 35 35 0 ],[0 28 28 0 0 ]);
      | fprintf('','COMMENT: end icon graphics');
      | fprintf('','COMMENT: begin icon text');
      | color('black');port_label('input',1,'d');
      | color('black');port_label('output',1,'q');
      | color('black');disp('\bf{z^{-1}}','texmode','on');
      | fprintf('','COMMENT: end icon text');
  Reinterpret : S-Function  LoadFcn=xlBlockLoadCallback(gcbh);  FunctionName=sysgen  Parameters=ptable_  mask(Xilinx Type Reinterpreter Block){infoedit=Changes signal type without altering the binary representation.   You can changed the signal between signed and unsigned, and relocate the binary point.<P><P>Hardware notes: In hardware this block costs nothing.<P><P>Example:  Suppose the input is 6 bits wide, signed, with 2 fractional bits, and the output is forced to unsigned with 0 fractional bits.  Then an input of -2.0 (1110.00 in binary 2's complement) becomes an output of 56 (111000 in binary)., force_arith_type_sgadvanced=, force_arith_type=on, arith_type_sgadvanced=, arith_type=Signed  (2's comp), force_bin_pt_sgadvanced=, force_bin_pt=on, bin_pt=15, has_advanced_control=0, sggui_pos=20,20,356,309, block_type=reinterpret, block_version=8.2, sg_icon_stat=45,20,1,1,white,blue,0,8982c1db, sg_mask_display=|, sg_list_contents=, sg_blockgui_xml=}
      mask sg_mask_display=|
      | fprintf('','COMMENT: begin icon graphics');
      | patch([0 45 45 0 ],[0 0 20 20 ],[0.77 0.82 0.91]);
      | patch([17 14 19 14 17 22 23 24 30 26 22 19 24 19 22 26 30 24 23 22 17 ],[2 5 10 15 18 18 17 18 18 14 18 15 10 5 2 6 2 2 3 2 2 ],[0.98 0.96 0.92]);
      | plot([0 0 45 45 0 ],[0 20 20 0 0 ]);
      | fprintf('','COMMENT: end icon graphics');
      | fprintf('','COMMENT: begin icon text');
      | color('black');disp('reinterpret');
      | fprintf('','COMMENT: end icon text');
      mask prompts: infoedit ""; force_arith_type_sgadvanced ""; force_arith_type "Force Arithmetic Type"; arith_type_sgadvanced ""; arith_type "Output Arithmetic Type"; force_bin_pt_sgadvanced ""; force_bin_pt "Force Binary Point"; bin_pt "Output Binary Point"; has_advanced_control ""; sggui_pos ""; block_type ""; block_version ""; sg_icon_stat ""; sg_mask_display ""; sg_list_contents ""; sg_blockgui_xml ""
      mask help:
      | Changes signal type without altering the binary representation.   You can changed the signal between signed and unsigned, and relocate the binary point.
      |
      | Hardware notes: In hardware this block costs nothing.
      |
      | Example:  Suppose the input is 6 bits wide, signed, with 2 fractional bits, and the output is forced to unsigned with 0 fractional bits.  Then an input of -2.0 (1110.00 in binary 2's complement) becomes an output of 56 (111000 in binary).
      mask init:
      | try
      |   tmp_gcb = gcb;
      |   tmp_gcbh = gcbh;
      |   xlMungeMaskParams;
      |   block_config = 'sysgen_blockset:Reinterpret_config';
      |   serialized_declarations = '{''arith_type''=>''Int'',''bin_pt''=>''Int'',''force_arith_type''=>''Bool'',''force_bin_pt''=>''Bool''}';
      |   ptable_ = xlblockprep(get_param(tmp_gcb, 'MaskWSVariables'));
      | catch
      |   global dbgsysgen;
      |   if(~isempty(dbgsysgen) && dbgsysgen)
      |     e = regexprep(lasterr, '\n', '\nError: ');
      |     disp(['Error: While running MaskInit code on block ' tmp_gcb ': ' e]);
      |     error(e);
      |   end
      | end
      settings: CopyFcn=xlBlockMoveCallback(gcbh);  DeleteFcn=xlDestroyGui(gcbh);  ModelCloseFcn=xlDestroyGui(gcbh);  PreSaveFcn=xlBlockPreSaveCallback(gcbh);  PostSaveFcn=xlBlockPostSaveCallback(gcbh);  DestroyFcn=xlDestroyGui(gcbh);  OpenFcn=xlOpenGui(gcbh, 'reinterpret_gui.xml', @reinterpretenablement, -1)  CloseFcn=xlDestroyGui(gcbh);  MoveFcn=xlBlockMoveCallback(gcbh);
      mask Help: eval('xlWeb(xlhtmldoclink(''Reinterpret''))');
      mask StyleString: edit,edit,checkbox,edit,popup(Unsigned|Signed  (2's comp)),edit,checkbox,edit,edit,edit,edit,edit,edit,edit,edit,edit
      mask Display:
      | fprintf('','COMMENT: begin icon graphics');
      | patch([0 45 45 0 ],[0 0 20 20 ],[0.77 0.82 0.91]);
      | patch([17 14 19 14 17 22 23 24 30 26 22 19 24 19 22 26 30 24 23 22 17 ],[2 5 10 15 18 18 17 18 18 14 18 15 10 5 2 6 2 2 3 2 2 ],[0.98 0.96 0.92]);
      | plot([0 0 45 45 0 ],[0 20 20 0 0 ]);
      | fprintf('','COMMENT: end icon graphics');
      | fprintf('','COMMENT: begin icon text');
      | color('black');disp('reinterpret');
      | fprintf('','COMMENT: end icon text');
  Reinterpret1 : S-Function  LoadFcn=xlBlockLoadCallback(gcbh);  FunctionName=sysgen  Parameters=ptable_  mask(Xilinx Type Reinterpreter Block){infoedit=Changes signal type without altering the binary representation.   You can changed the signal between signed and unsigned, and relocate the binary point.<P><P>Hardware notes: In hardware this block costs nothing.<P><P>Example:  Suppose the input is 6 bits wide, signed, with 2 fractional bits, and the output is forced to unsigned with 0 fractional bits.  Then an input of -2.0 (1110.00 in binary 2's complement) becomes an output of 56 (111000 in binary)., force_arith_type_sgadvanced=, force_arith_type=on, arith_type_sgadvanced=, arith_type=Signed  (2's comp), force_bin_pt_sgadvanced=, force_bin_pt=on, bin_pt=15, has_advanced_control=0, sggui_pos=20,20,356,309, block_type=reinterpret, block_version=8.2, sg_icon_stat=45,20,1,1,white,blue,0,8982c1db, sg_mask_display=|, sg_list_contents=, sg_blockgui_xml=}
      mask sg_mask_display=|
      | fprintf('','COMMENT: begin icon graphics');
      | patch([0 45 45 0 ],[0 0 20 20 ],[0.77 0.82 0.91]);
      | patch([17 14 19 14 17 22 23 24 30 26 22 19 24 19 22 26 30 24 23 22 17 ],[2 5 10 15 18 18 17 18 18 14 18 15 10 5 2 6 2 2 3 2 2 ],[0.98 0.96 0.92]);
      | plot([0 0 45 45 0 ],[0 20 20 0 0 ]);
      | fprintf('','COMMENT: end icon graphics');
      | fprintf('','COMMENT: begin icon text');
      | color('black');disp('reinterpret');
      | fprintf('','COMMENT: end icon text');
      mask prompts: infoedit ""; force_arith_type_sgadvanced ""; force_arith_type "Force Arithmetic Type"; arith_type_sgadvanced ""; arith_type "Output Arithmetic Type"; force_bin_pt_sgadvanced ""; force_bin_pt "Force Binary Point"; bin_pt "Output Binary Point"; has_advanced_control ""; sggui_pos ""; block_type ""; block_version ""; sg_icon_stat ""; sg_mask_display ""; sg_list_contents ""; sg_blockgui_xml ""
      mask help:
      | Changes signal type without altering the binary representation.   You can changed the signal between signed and unsigned, and relocate the binary point.
      |
      | Hardware notes: In hardware this block costs nothing.
      |
      | Example:  Suppose the input is 6 bits wide, signed, with 2 fractional bits, and the output is forced to unsigned with 0 fractional bits.  Then an input of -2.0 (1110.00 in binary 2's complement) becomes an output of 56 (111000 in binary).
      mask init: same as warplab_mimo_4x4/Radio_1_Outputs/Reinterpret
      settings: CopyFcn=xlBlockMoveCallback(gcbh);  DeleteFcn=xlDestroyGui(gcbh);  ModelCloseFcn=xlDestroyGui(gcbh);  PreSaveFcn=xlBlockPreSaveCallback(gcbh);  PostSaveFcn=xlBlockPostSaveCallback(gcbh);  DestroyFcn=xlDestroyGui(gcbh);  OpenFcn=xlOpenGui(gcbh, 'reinterpret_gui.xml', @reinterpretenablement, -1)  CloseFcn=xlDestroyGui(gcbh);  MoveFcn=xlBlockMoveCallback(gcbh);
      mask Help: eval('xlWeb(xlhtmldoclink(''Reinterpret''))');
      mask StyleString: edit,edit,checkbox,edit,popup(Unsigned|Signed  (2's comp)),edit,checkbox,edit,edit,edit,edit,edit,edit,edit,edit,edit
      mask Display:
      | fprintf('','COMMENT: begin icon graphics');
      | patch([0 45 45 0 ],[0 0 20 20 ],[0.77 0.82 0.91]);
      | patch([17 14 19 14 17 22 23 24 30 26 22 19 24 19 22 26 30 24 23 22 17 ],[2 5 10 15 18 18 17 18 18 14 18 15 10 5 2 6 2 2 3 2 2 ],[0.98 0.96 0.92]);
      | plot([0 0 45 45 0 ],[0 20 20 0 0 ]);
      | fprintf('','COMMENT: end icon graphics');
      | fprintf('','COMMENT: begin icon text');
      | color('black');disp('reinterpret');
      | fprintf('','COMMENT: end icon text');
  Terminator1 : Terminator
  Terminator2 : Terminator
  wires:
  Register1/1 -> Radio_1_DAC_Q/1(Q)
  Register/1 -> Radio_1_DAC_I/1(I)
  16MSB/1 -> Reinterpret/1
  16LSB/1 -> Reinterpret1/1
  Reinterpret/1 -> Register/1
  Reinterpret1/1 -> Register1/1
  Radio_1_DAC_I/1(I_out) -> Terminator1/1
  Radio_1_DAC_Q/1(Q_out) -> Terminator2/1
  32b/1 -> 16LSB/1, 16MSB/1
